simulink model "SquareCartesian_backup"  (R2017b)
settings: Solver=VariableStepAuto  StartTime=0.0  StopTime=50  RelTol=1e-3
PreLoadFcn:
  | config_parameters
model workspace (MAT data in the model file):
  r = 0.11
undefined symbols (not defined in the file): b, sampleTime, X, Y, Z
libraries: sm_lib x127, nesl_utility x20, fl_lib x8, vrlib x4, mobileRoboticsLib x2, simulink x1
(part 1 of 4)
settings Model: Creator=ty  LastModifiedBy=ty
settings DataIOCC: ExternalInput=[r, b]
settings SimMechanicsCC: VisOnUpdateDiagram=on  VisDuringSimulation=on

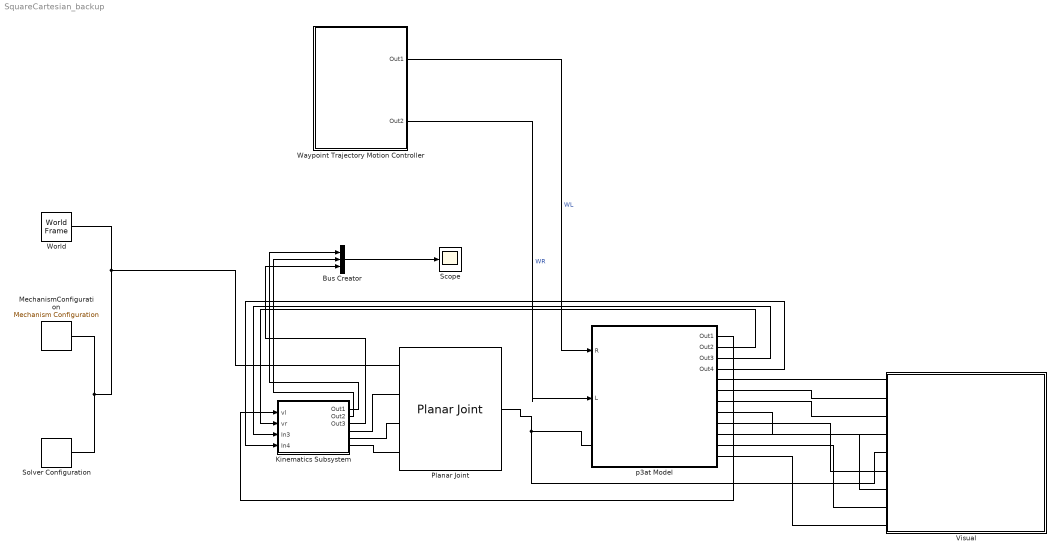
== system SquareCartesian_backup ==
  Bus Creator : BusCreator  Inputs=3
  Kinematics Subsystem : Subsystem
  MechanismConfiguration : sm_lib/Utilities/Mechanism Configuration  UniformGravity=Constant  GravityVector=[0 0 -9.80665]  GravityUnits=m/s^2  LinearizationDelta=0.001
  Planar Joint : sm_lib/Joints/Planar Joint  SenseConstraintForce=off  SenseConstraintForceX=off  SenseConstraintForceY=off  SenseConstraintForceZ=off  SenseConstraintTorque=off  SenseConstraintTorqueX=off  SenseConstraintTorqueY=off  SenseConstraintTorqueZ=off  SenseTotalForce=off  SenseTotalForceX=off  SenseTotalForceY=off  SenseTotalForceZ=off  SenseTotalTorque=off  SenseTotalTorqueX=off  SenseTotalTorqueY=off  SenseTotalTorqueZ=off  CompositeWrenchDir=FollowerOnBase  CompositeWrenchFrame=BaseFrame  PxEquilibriumPosition=0  PxEquilibriumPositionUnits=m  PxSpringStiffness=0  PxSpringStiffnessUnits=N/m  PxDampingCoefficient=0  PxDampingCoefficientUnits=N/(m/s)  PxTorqueActuationMode=ComputedTorque  PxMotionActuationMode=InputMotion  PxSensePosition=off  PxSenseVelocity=off  PxSenseAcceleration=off  PxSenseTorqueForce=off  PxPositionTargetSpecify=on  PxPositionTargetPriority=High  PxPositionTargetValue=0  PxPositionTargetValueUnits=m  PxVelocityTargetSpecify=off  PxVelocityTargetPriority=High  PxVelocityTargetValue=0  PxVelocityTargetValueUnits=m/s  PyEquilibriumPosition=0  PyEquilibriumPositionUnits=m  PySpringStiffness=0  PySpringStiffnessUnits=N/m  PyDampingCoefficient=0  PyDampingCoefficientUnits=N/(m/s)  PyTorqueActuationMode=ComputedTorque  PyMotionActuationMode=InputMotion  PySensePosition=off  PySenseVelocity=off  PySenseAcceleration=off  PySenseTorqueForce=off  PyPositionTargetSpecify=on  PyPositionTargetPriority=High  PyPositionTargetValue=0  PyPositionTargetValueUnits=m  PyVelocityTargetSpecify=off  PyVelocityTargetPriority=High  PyVelocityTargetValue=0  PyVelocityTargetValueUnits=m/s  RzEquilibriumPosition=0  RzEquilibriumPositionUnits=deg  RzSpringStiffness=0  RzSpringStiffnessUnits=N*m/deg  RzDampingCoefficient=0  RzDampingCoefficientUnits=N*m/(deg/s)  RzTorqueActuationMode=ComputedTorque  RzMotionActuationMode=InputMotion  RzSensePosition=off  RzSenseVelocity=off  RzSenseAcceleration=off  RzSenseTorqueForce=off  RzPositionTargetSpecify=on  RzPositionTargetPriority=High  RzPositionTargetValue=0  RzPositionTargetValueUnits=deg  RzVelocityTargetSpecify=off  RzVelocityTargetPriority=High  RzVelocityTargetValue=0  RzVelocityTargetValueUnits=deg/s
  Scope : Scope
  Solver Configuration : nesl_utility/Solver Configuration  PhysicalDomain=network_engine_domain  SubClassName=solver  LeftPortType=input  RightPortType=generic  Accelerate=off  Tones=[]  Harmonics=[]  SimulateNoise=off  Profile=off  UseLocalSampling=off  EnableSwitchedLinearOptims=on  FrequencyDomain=off  UseCCode=off  RelTol=0.001  AbsTol=1e-06  MinStep=1e-09  ToWorkspace=off  RevertToSquareIcSolve=off  NumHomotopyIterations=100  PhasorMode=off  PhasorModeNumHarmonics=1  DoDC=off  ResidualTolerance=1e-09  UseLocalSolver=off  LocalSolverChoice=NE_BACKWARD_EULER_ADVANCER  LocalSolverSampleTime=0.001  DoFixedCost=off  MaxNonlinIter=3  MaxModeIter=2  LinearAlgebra=Sparse  DelaysMemoryBudget=1024  AutomaticFiltering=on  FilteringTimeConstant=0.001
  Visual : Subsystem
  Waypoint Trajectory Motion Controller : Subsystem
  World : sm_lib/Frames and Transforms/World Frame
  p3at Model : Subsystem
  wires:
  p3at Model/1(Out1) -> Kinematics Subsystem/1(vl)
  p3at Model/2(Out2) -> Kinematics Subsystem/2(vr)
  p3at Model/3(Out3) -> Kinematics Subsystem/3(In3)
  p3at Model/4(Out4) -> Kinematics Subsystem/4(In4)
  Kinematics Subsystem/1(Out1) -> Bus Creator/1
  Kinematics Subsystem/2(Out2) -> Bus Creator/2
  Kinematics Subsystem/3(Out3) -> Bus Creator/3
  Bus Creator/1 -> Scope/1
  Waypoint Trajectory Motion Controller/1(Out1) -> p3at Model/1(R)  "WL"
  Waypoint Trajectory Motion Controller/2(Out2) -> p3at Model/2(L)  "WR"
  connections:
  MechanismConfiguration/RConn1 -- Planar Joint/LConn1 -- World/RConn1 -- Solver Configuration/RConn1
  Planar Joint/LConn4 -- Kinematics Subsystem/RConn3
  Kinematics Subsystem/RConn2 -- Planar Joint/LConn3
  Kinematics Subsystem/RConn1 -- Planar Joint/LConn2
  Planar Joint/RConn1 -- Visual/LConn5 -- p3at Model/LConn1
  p3at Model/RConn1 -- Visual/LConn1
  Visual/LConn2 -- p3at Model/RConn2
  Visual/LConn3 -- p3at Model/RConn3
  Visual/LConn4 -- p3at Model/RConn4
  Visual/LConn6 -- p3at Model/RConn5
  Visual/LConn7 -- p3at Model/RConn6
  Visual/LConn8 -- p3at Model/RConn7
  Visual/LConn9 -- p3at Model/RConn8

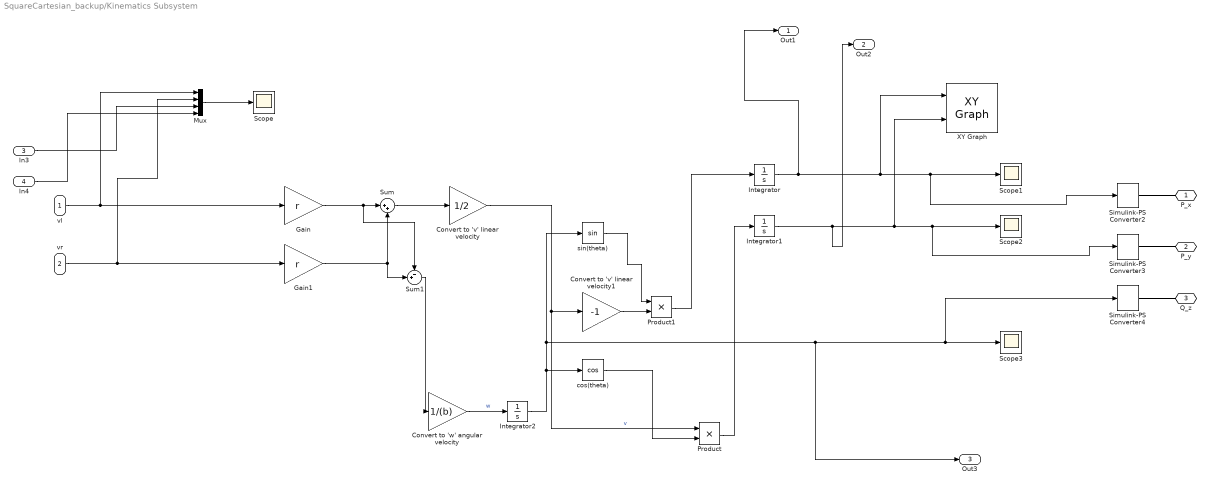
== system SquareCartesian_backup/Kinematics Subsystem ==
  vl : Inport
  vr : Inport  Port=2
  In3 : Inport  Port=3
  In4 : Inport  Port=4
  Convert to 'v' linear velocity : Gain  Gain=1/2
  Convert to 'v' linear velocity1 : Gain  Gain=-1
  Convert to 'w' angular velocity : Gain  Gain=1/(b)
  Gain : Gain  Gain=r
  Gain1 : Gain  Gain=r
  Integrator : Integrator
  Integrator1 : Integrator
  Integrator2 : Integrator
  Mux : Mux
  Product : Product
  Product1 : Product
  Scope{,1..3} (4 alike) : Scope
  Simulink-PS Converter2 : nesl_utility/Simulink-PS Converter  PhysicalDomain=network_engine_domain  SubClassName=ps_input  LeftPortType=input  RightPortType=output  PseudoPeriodic=off  Frequencies=[]  NoiseDistribution=none  NoiseParameters=[]  Unit=1  AffineConversion=off  FilteringAndDerivatives=filter  SimscapeFilterOrder=2  InputFilterTimeConstant=0.01  UdotUserProvided=1
  Simulink-PS Converter3 : nesl_utility/Simulink-PS Converter  PhysicalDomain=network_engine_domain  SubClassName=ps_input  LeftPortType=input  RightPortType=output  PseudoPeriodic=off  Frequencies=[]  NoiseDistribution=none  NoiseParameters=[]  Unit=1  AffineConversion=off  FilteringAndDerivatives=filter  SimscapeFilterOrder=2  InputFilterTimeConstant=0.01  UdotUserProvided=1
  Simulink-PS Converter4 : nesl_utility/Simulink-PS Converter  PhysicalDomain=network_engine_domain  SubClassName=ps_input  LeftPortType=input  RightPortType=output  PseudoPeriodic=off  Frequencies=[]  NoiseDistribution=none  NoiseParameters=[]  Unit=1  AffineConversion=off  FilteringAndDerivatives=filter  SimscapeFilterOrder=2  InputFilterTimeConstant=0.01  UdotUserProvided=1
  Sum : Sum  Inputs=|++
  Sum1 : Sum  Inputs=-+|
  XY Graph : simulink/Sinks/XY Graph  xmin=-10  xmax=10  ymin=-10  ymax=10  st=.05
  cos(theta) : Trigonometry  Operator=cos
  sin(theta) : Trigonometry
  P_x : PMIOPort  Port=1  Side=Right
  P_y : PMIOPort  Port=2  Side=Right
  Q_z : PMIOPort  Port=3  Side=Right
  Out1 : Outport
  Out2 : Outport  Port=2
  Out3 : Outport  Port=3
  wires:
  Convert to 'v' linear velocity1/1 -> Product1/2
  Mux/1 -> Scope/1
  Product/1 -> Integrator1/1
  Product1/1 -> Integrator/1
  vr/1 -> Gain1/1, Mux/2
  vl/1 -> Gain/1, Mux/1
  Convert to 'v' linear velocity/1 -> Product/1, Convert to 'v' linear velocity1/1  "v"
  Sum1/1 -> Convert to 'w' angular velocity/1
  cos(theta)/1 -> Product/2
  sin(theta)/1 -> Product1/1
  Convert to 'w' angular velocity/1 -> Integrator2/1  "w"
  Integrator/1 -> Out1/1, XY Graph/1, Scope1/1, Simulink-PS Converter2/1
  Sum/1 -> Convert to 'v' linear velocity/1
  Gain/1 -> Sum/1, Sum1/1
  Gain1/1 -> Sum1/2, Sum/2
  In3/1 -> Mux/3
  In4/1 -> Mux/4
  Integrator1/1 -> Out2/1, XY Graph/2, Scope2/1, Simulink-PS Converter3/1
  Integrator2/1 -> cos(theta)/1, Scope3/1, Simulink-PS Converter4/1, Out3/1, sin(theta)/1
  connections:
  Simulink-PS Converter3/RConn1 -- P_y/RConn1
  Simulink-PS Converter2/RConn1 -- P_x/RConn1
  Simulink-PS Converter4/RConn1 -- Q_z/RConn1

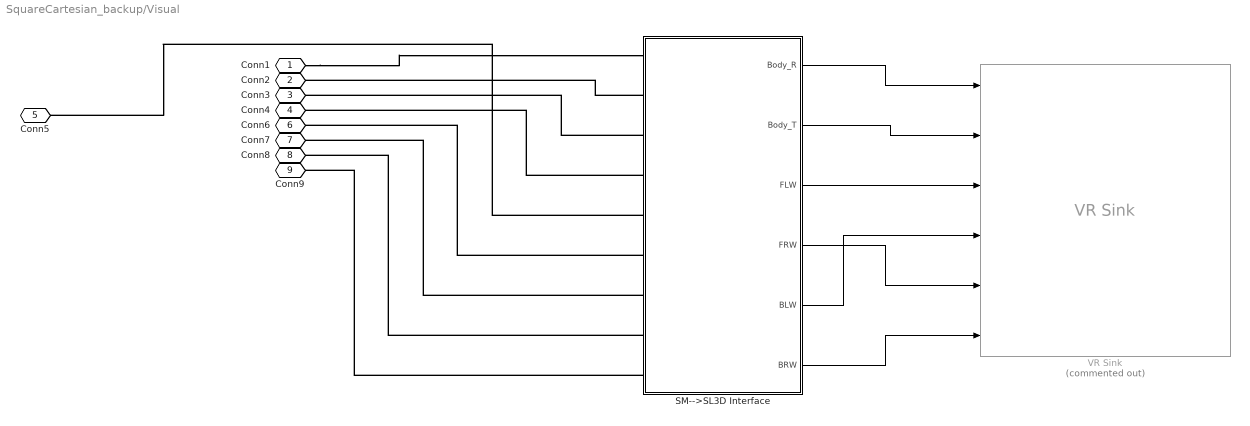
== system SquareCartesian_backup/Visual ==
  SM-->SL3D Interface : Subsystem
  VR Sink : vrlib/VR Sink  Commented=on  InstantiateOnLoad=on  SampleTime=0.1  ViewEnable=on  RemoteChange=off  RemoteView=off  FieldsWritten=URDF_p3original_Transform.rotation.4.1.1.double#URDF_p3original_Transform.translation.3.1.1.double#joint_base_front_left_axle_joint.rotation.4.1.1.double#joint_p3at_back_left_axle_joint.rotation.4.1.1.double#joint_base_front_right_axle_joint.rotation.4.1.1.double#joint_p3at_back_right_axle_joint.rotation.4.1.1.double  WorldFileName=/home/ty/Matlab UGV Simulations/Environments/p3atEnv.wrl  WorldDescription=Pioneer3at Model  AutoView=off  VideoDimensions=[]  AllowVariableSize=off
      settings: SourceProductBaseCode=VR
  Conn1 : PMIOPort  Port=1  Side=Left
  Conn2 : PMIOPort  Port=2  Side=Left
  Conn3 : PMIOPort  Port=3  Side=Left
  Conn4 : PMIOPort  Port=4  Side=Left
  Conn5 : PMIOPort  Port=5  Side=Left
  Conn6 : PMIOPort  Port=6  Side=Left
  Conn7 : PMIOPort  Port=7  Side=Left
  Conn8 : PMIOPort  Port=8  Side=Left
  Conn9 : PMIOPort  Port=9  Side=Left
  wires:
  SM-->SL3D Interface/1(Body_R) -> VR Sink/1
  SM-->SL3D Interface/2(Body_T) -> VR Sink/2
  SM-->SL3D Interface/3(FLW) -> VR Sink/3
  SM-->SL3D Interface/4(FRW) -> VR Sink/5
  SM-->SL3D Interface/5(BLW) -> VR Sink/4
  SM-->SL3D Interface/6(BRW) -> VR Sink/6
  connections:
  SM-->SL3D Interface/LConn5 -- Conn5/RConn1
  SM-->SL3D Interface/LConn3 -- Conn3/RConn1
  Conn1/RConn1 -- SM-->SL3D Interface/LConn1
  SM-->SL3D Interface/LConn7 -- Conn7/RConn1
  SM-->SL3D Interface/LConn2 -- Conn2/RConn1
  SM-->SL3D Interface/LConn6 -- Conn6/RConn1
  SM-->SL3D Interface/LConn8 -- Conn8/RConn1
  SM-->SL3D Interface/LConn4 -- Conn4/RConn1
  SM-->SL3D Interface/LConn9 -- Conn9/RConn1

== system SquareCartesian_backup/Waypoint Trajectory Motion Controller ==
  Differential Drive Inverse Kinematics : Subsystem  AncestorBlock=mobileRoboticsLib/Kinematic Models/Differential Drive/Differential Drive Inverse Kinematics  mask(Differential Drive Inverse Kinematics){wheelRadius=r, wheelBase=b}
      mask prompts: wheelRadius "Wheel Radius [m]"; wheelBase "Wheelbase [m]"
      mask help:
      | Calculates the forward kinematics for a differential drive vehicle.
      |
      | Input: [v; w], the linear (m/s) and angular (rad/s) velocities of the vehicle
      |
      | Output: [wL; wR], the left and right wheel speeds (rad/s)
      mask Help: web('matlab:edit mrsDocDifferentialDrive')
  Differential Drive Simulation : mobileRoboticsLib/Kinematic Models/Differential Drive/Differential Drive Simulation  OverrideUsingVariant=mode==2  wheelRadius=r  wheelBase=b  initX=0  initY=0  initAngle=0  Ts=sampleTime
      settings: SourceProductName=Mobile Robotics Simulation Library
  Mux : Mux  Inputs=2
  Robot Visualizer : mobileRoboticsLib/Environments/Robot Visualizer  Priority=99  robotRadius=.25  showTrajectory=on  hasWaypoints=on  hasLidar=off  sensorOffset=[ 0 0 ]  scanAngles=0  hasObjDetector=off  objDetectorOffset=[ 0, 0 ]  objDetectorAngle=0  objDetectorFOV=0  objDetectorMaxRange=0  objectColors=0  objectMarkers='s'
      settings: SourceProductName=Ground Vehicles Library
  Waypoint Tracking Logic : Stateflow chart  TreatAsAtomicUnit=on
  Waypoints1 : Constant  Value=[0,0; 2,2; -2,2; -2,-2; 2,-2; 2,2; 0,0]
  Out1 : Outport
  Out2 : Outport  Port=2
  wires:
  Differential Drive Inverse Kinematics/3(WR) -> Out1/1
  Differential Drive Inverse Kinematics/2(WL) -> Out2/1
  Differential Drive Simulation/1 -> Waypoint Tracking Logic/1(pose), Robot Visualizer/1  "pose"
  Waypoint Tracking Logic/2(w) -> Mux/2  "w"
  Mux/1 -> Differential Drive Inverse Kinematics/1(vRef)  "vRef"
  Waypoint Tracking Logic/1(v) -> Mux/1  "v"
  Waypoints1/1 -> Robot Visualizer/2, Waypoint Tracking Logic/2(waypoints)
  Differential Drive Inverse Kinematics/1(wheelSpd) -> Differential Drive Simulation/1  "wheelSpeeds"

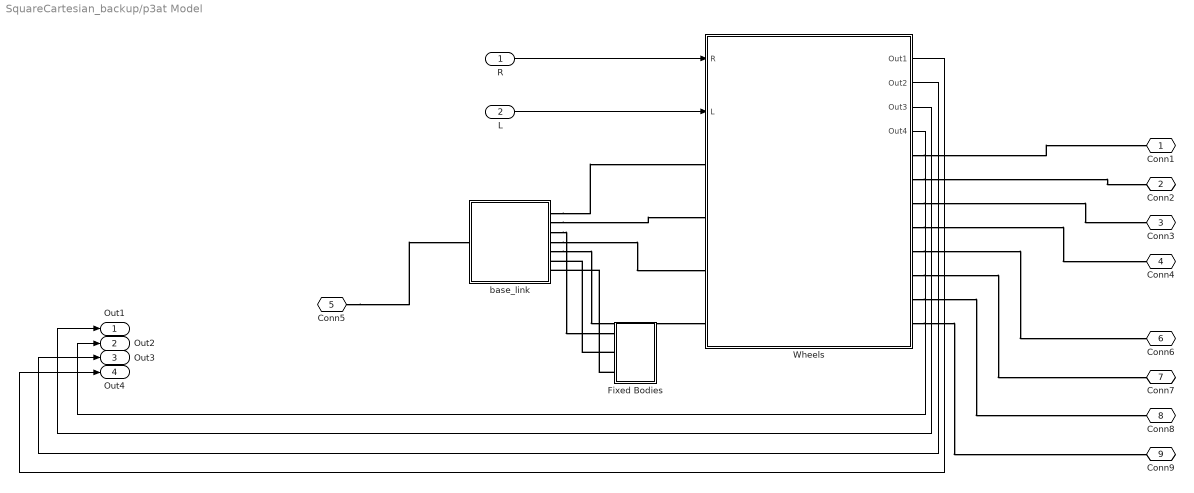
== system SquareCartesian_backup/p3at Model ==
  R : Inport
  L : Inport  Port=2
  Fixed Bodies : Subsystem
  Wheels : Subsystem
  base_link : Subsystem
  Conn1 : PMIOPort  Port=1  Side=Right
  Conn2 : PMIOPort  Port=2  Side=Right
  Conn3 : PMIOPort  Port=3  Side=Right
  Conn4 : PMIOPort  Port=4  Side=Right
  Conn5 : PMIOPort  Port=5  Side=Left
  Conn6 : PMIOPort  Port=6  Side=Right
  Conn7 : PMIOPort  Port=7  Side=Right
  Conn8 : PMIOPort  Port=8  Side=Right
  Conn9 : PMIOPort  Port=9  Side=Right
  Out1 : Outport
  Out2 : Outport  Port=2
  Out3 : Outport  Port=3
  Out4 : Outport  Port=4
  wires:
  Wheels/3(Out3) -> Out1/1
  Wheels/4(Out4) -> Out2/1
  Wheels/2(Out2) -> Out3/1
  Wheels/1(Out1) -> Out4/1
  R/1 -> Wheels/1(R)
  L/1 -> Wheels/2(L)
  connections:
  Conn5/RConn1 -- base_link/LConn1
  base_link/RConn3 -- Fixed Bodies/LConn1
  Fixed Bodies/LConn2 -- base_link/RConn6
  Fixed Bodies/LConn3 -- base_link/RConn7
  Wheels/RConn1 -- Conn1/RConn1
  Wheels/RConn2 -- Conn2/RConn1
  Wheels/RConn3 -- Conn3/RConn1
  Wheels/RConn4 -- Conn4/RConn1
  Wheels/RConn5 -- Conn6/RConn1
  base_link/RConn1 -- Wheels/LConn1
  base_link/RConn2 -- Wheels/LConn2
  Wheels/RConn6 -- Conn7/RConn1
  base_link/RConn4 -- Wheels/LConn3
  base_link/RConn5 -- Wheels/LConn4
  Wheels/RConn7 -- Conn8/RConn1
  Wheels/RConn8 -- Conn9/RConn1

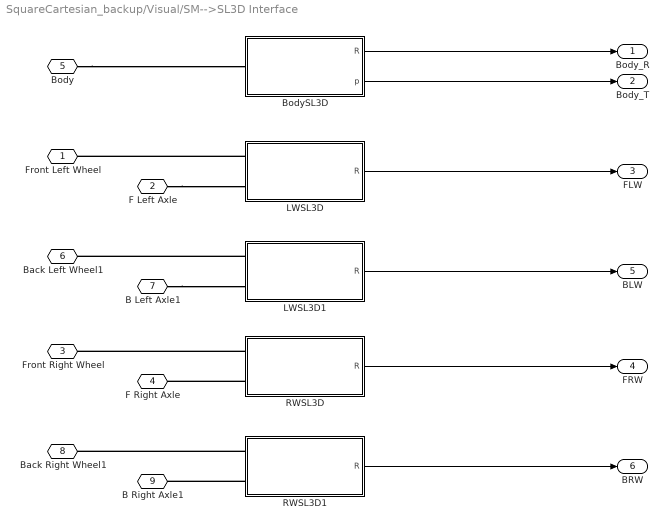
== system SquareCartesian_backup/Visual/SM-->SL3D Interface ==
  "BodySL3D " : Subsystem
  LWSL3D : Subsystem
  LWSL3D1 : Subsystem
  RWSL3D : Subsystem
  RWSL3D1 : Subsystem
  Front Left Wheel : PMIOPort  Port=1  Side=Left
  F Left Axle : PMIOPort  Port=2  Side=Left
  Front Right Wheel : PMIOPort  Port=3  Side=Left
  F Right Axle : PMIOPort  Port=4  Side=Left
  Body : PMIOPort  Port=5  Side=Left
  Back Left Wheel1 : PMIOPort  Port=6  Side=Left
  B Left Axle1 : PMIOPort  Port=7  Side=Left
  Back Right Wheel1 : PMIOPort  Port=8  Side=Left
  B Right Axle1 : PMIOPort  Port=9  Side=Left
  Body_R : Outport
  Body_T : Outport  Port=2
  FLW : Outport  Port=3
  FRW : Outport  Port=4
  BLW : Outport  Port=5
  BRW : Outport  Port=6
  wires:
  "BodySL3D "/1(R) -> Body_R/1
  "BodySL3D "/2(p) -> Body_T/1
  RWSL3D/1(R) -> FRW/1
  LWSL3D/1(R) -> FLW/1
  LWSL3D1/1(R) -> BLW/1
  RWSL3D1/1(R) -> BRW/1
  connections:
  RWSL3D/LConn2 -- F Right Axle/RConn1
  F Left Axle/RConn1 -- LWSL3D/LConn2
  Body/RConn1 -- "BodySL3D "/LConn1
  RWSL3D/LConn1 -- Front Right Wheel/RConn1
  LWSL3D/LConn1 -- Front Left Wheel/RConn1
  B Left Axle1/RConn1 -- LWSL3D1/LConn2
  LWSL3D1/LConn1 -- Back Left Wheel1/RConn1
  RWSL3D1/LConn1 -- Back Right Wheel1/RConn1
  RWSL3D1/LConn2 -- B Right Axle1/RConn1

== system SquareCartesian_backup/Waypoint Trajectory Motion Controller/Differential Drive Inverse Kinematics ==
  vRef : Inport
  Demux : Demux  Outputs=2
  MATLAB Function : MATLAB Function  TreatAsAtomicUnit=on
  Mux : Mux  Inputs=2
  wheelSpd : Outport
  WL : Outport  Port=2
  WR : Outport  Port=3
  wires:
  MATLAB Function/1(wL) -> WL/1, Mux/1  "wL"
  MATLAB Function/2(wR) -> WR/1, Mux/2  "wR"
  Mux/1 -> wheelSpd/1
  vRef/1 -> Demux/1
  Demux/1 -> MATLAB Function/1(v)  "v"
  Demux/2 -> MATLAB Function/2(w)  "w"

== system SquareCartesian_backup/p3at Model/Fixed Bodies ==
  Sonar Arrays : Subsystem
  Top Plate : Subsystem
  Conn1 : PMIOPort  Port=1  Side=Left
  Conn2 : PMIOPort  Port=2  Side=Left
  Conn3 : PMIOPort  Port=3  Side=Left
  connections:
  Conn1/RConn1 -- Top Plate/LConn1
  Sonar Arrays/LConn1 -- Conn2/RConn1
  Sonar Arrays/LConn2 -- Conn3/RConn1

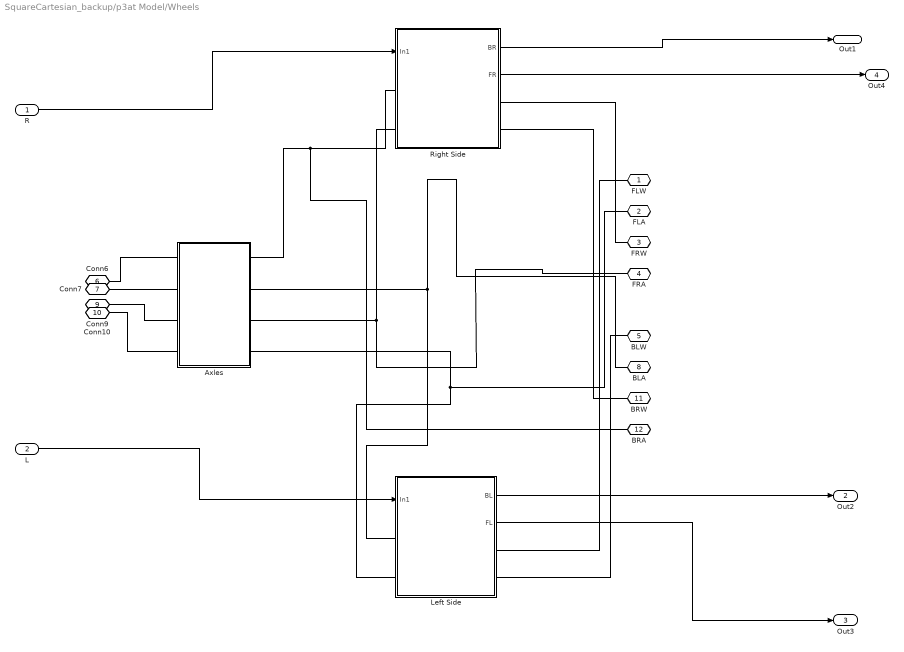
== system SquareCartesian_backup/p3at Model/Wheels ==
  R : Inport
  L : Inport  Port=2
  Axles : Subsystem
  Left Side : Subsystem
  Right Side : Subsystem
  FLW : PMIOPort  Port=1  Side=Right
  FLA : PMIOPort  Port=2  Side=Right
  FRW : PMIOPort  Port=3  Side=Right
  FRA : PMIOPort  Port=4  Side=Right
  BLW : PMIOPort  Port=5  Side=Right
  Conn6 : PMIOPort  Port=6  Side=Left
  Conn7 : PMIOPort  Port=7  Side=Left
  BLA : PMIOPort  Port=8  Side=Right
  Conn9 : PMIOPort  Port=9  Side=Left
  Conn10 : PMIOPort  Port=10  Side=Left
  BRW : PMIOPort  Port=11  Side=Right
  BRA : PMIOPort  Port=12  Side=Right
  Out1 : Outport
  Out2 : Outport  Port=2
  Out3 : Outport  Port=3
  Out4 : Outport  Port=4
  wires:
  R/1 -> Right Side/1(In1)
  Right Side/1(BR) -> Out1/1
  Right Side/2(FR) -> Out4/1
  L/1 -> Left Side/1(In1)
  Left Side/1(BL) -> Out2/1
  Left Side/2(FL) -> Out3/1
  connections:
  FLA/RConn1 -- Left Side/LConn2 -- Axles/RConn4
  FRA/RConn1 -- Axles/RConn3 -- Right Side/LConn2
  BLA/RConn1 -- Left Side/LConn1 -- Axles/RConn2
  Conn6/RConn1 -- Axles/LConn1
  Conn7/RConn1 -- Axles/LConn2
  Axles/LConn3 -- Conn9/RConn1
  Axles/LConn4 -- Conn10/RConn1
  Axles/RConn1 -- Right Side/LConn1 -- BRA/RConn1
  FRW/RConn1 -- Right Side/RConn1
  BRW/RConn1 -- Right Side/RConn2
  Left Side/RConn1 -- FLW/RConn1
  BLW/RConn1 -- Left Side/RConn2

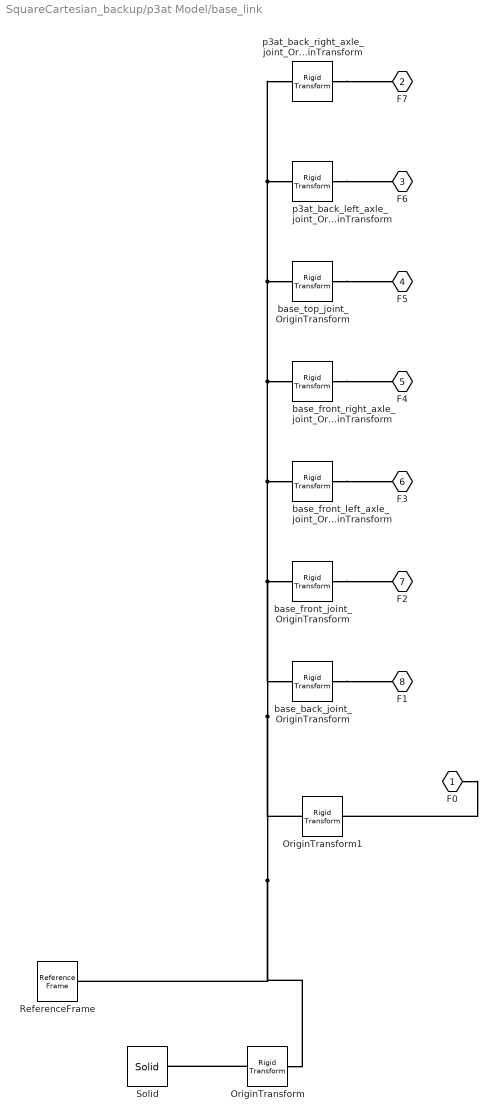
== system SquareCartesian_backup/p3at Model/base_link ==
  OriginTransform : sm_lib/Frames and Transforms/Rigid Transform  TranslationMethod=Cartesian  TranslationStandardOffset=0  TranslationLengthUnit=m  TranslationStandardAxis=+Z  TranslationCartesianOffset=[0, 0, -0.177]  TranslationROffset=0  TranslationROffsetUnits=m  TranslationZOffset=0  TranslationZOffsetUnits=m  TranslationThetaOffset=0  TranslationThetaOffsetUnits=deg  RotationMethod=RotationSequence  RotationAngleUnits=deg  RotationStandardAxis=+Z  RotationAngle=0.0  RotationArbitraryAxis=[0 0 1]  FollAlignAxisA=+X  BaseAlignAxisA=+Y  FollAlignAxisB=+Y  BaseAlignAxisB=+Z  RotationSequenceAxes=BaseAxes  RotationSequence=XYZ  RotationSequenceAngles=[0, 0, 0]  RotationSequenceAnglesUnits=rad  RotationMatrix=[1 0 0; 0 1 0; 0 0 1]
  OriginTransform1 : sm_lib/Frames and Transforms/Rigid Transform  TranslationMethod=Cartesian  TranslationStandardOffset=0  TranslationLengthUnit=m  TranslationStandardAxis=+Z  TranslationCartesianOffset=[0, 0, -0.177]  TranslationROffset=0  TranslationROffsetUnits=m  TranslationZOffset=0  TranslationZOffsetUnits=m  TranslationThetaOffset=0  TranslationThetaOffsetUnits=deg  RotationMethod=StandardAxis  RotationAngleUnits=deg  RotationStandardAxis=+Z  RotationAngle=90.0  RotationArbitraryAxis=[0 0 1]  FollAlignAxisA=+X  BaseAlignAxisA=+Y  FollAlignAxisB=+Y  BaseAlignAxisB=+Z  RotationSequenceAxes=BaseAxes  RotationSequence=XYZ  RotationSequenceAngles=[0, 0, 0]  RotationSequenceAnglesUnits=rad  RotationMatrix=[1 0 0; 0 1 0; 0 0 1]
  ReferenceFrame : sm_lib/Frames and Transforms/Reference Frame
  Solid : sm_lib/Body Elements/Solid  InertiaType=Custom  Mass=21.5  MassUnits=kg  CenterOfMass=[0, 0, 0]  CenterOfMassUnits=m  MomentsOfInertia=[0.3338, 0.4783, 0.3338]  MomentsOfInertiaUnits=kg*m^2  ProductsOfInertia=[0, 0, 0]  ProductsOfInertiaUnits=kg*m^2  DensityBased=on  Density=1000  DensityUnits=kg/(m^3)  DoExposeReferenceFrame=on  SerializedFrames=<Frames/>  GraphicType=FromGeometry  MarkerShape=Sphere  MarkerSize=10  MarkerSizeUnits=m  GraphicVisPropType=SimpleVisualProperties  GraphicDiffuseColor=[0.851, 0, 0]  GraphicSpecularColor=[0.5 0.5 0.5 1.0]  GraphicAmbientColor=[0.15 0.15 0.15 1.0]  GraphicEmissiveColor=[0.0 0.0 0.0 1.0]  GraphicShininess=75  GraphicOpacity=1  GeometryShape=FromFile  RectangleSize=[1 1]  RectangleSizeUnits=m  BrickDimensions=[1 1 1]  BrickDimensionUnits=m  CylinderRadius=1  CylinderRadiusUnits=m  CylinderLength=1  CylinderLengthUnits=m  SphereRadius=1  SphereRadiusUnits=m  EllipsoidRadii=[1 1 1]  EllipsoidRadiiUnits=m  ExtrusionCrossSection=[1 1; -1 1; -1 -1; 1 -1]  ExtrusionCrossSectionUnits=m  ExtrusionLength=1  ExtrusionLengthUnits=m  PolygonNumSides=3  PolygonOuterRadius=1  PolygonOuterRadiusUnits=m  ExtGeomFileType=STL  ExtGeomFileName=/home/ty/Matlab UGV Simulations/Models/p3at_meshes/chassis.stl  ExtGeomFileUnits=m  RevolutionCrossSection=[1 1; 1 -1; 2 -1; 2 1]  RevolutionCrossSectionUnits=m  RevolutionExtent=Full  RevolutionAngle=180  RevolutionAngleUnits=deg
  base_back_joint_OriginTransform : sm_lib/Frames and Transforms/Rigid Transform  TranslationMethod=Cartesian  TranslationStandardOffset=0  TranslationLengthUnit=m  TranslationStandardAxis=+Z  TranslationCartesianOffset=[-0.187, 0, 0.247]  TranslationROffset=0  TranslationROffsetUnits=m  TranslationZOffset=0  TranslationZOffsetUnits=m  TranslationThetaOffset=0  TranslationThetaOffsetUnits=deg  RotationMethod=RotationSequence  RotationAngleUnits=deg  RotationStandardAxis=+Z  RotationAngle=0.0  RotationArbitraryAxis=[0 0 1]  FollAlignAxisA=+X  BaseAlignAxisA=+Y  FollAlignAxisB=+Y  BaseAlignAxisB=+Z  RotationSequenceAxes=BaseAxes  RotationSequence=XYZ  RotationSequenceAngles=[0, 0, 0]  RotationSequenceAnglesUnits=rad  RotationMatrix=[1 0 0; 0 1 0; 0 0 1]
  base_front_joint_OriginTransform : sm_lib/Frames and Transforms/Rigid Transform  TranslationMethod=Cartesian  TranslationStandardOffset=0  TranslationLengthUnit=m  TranslationStandardAxis=+Z  TranslationCartesianOffset=[0.193, 0, 0.25]  TranslationROffset=0  TranslationROffsetUnits=m  TranslationZOffset=0  TranslationZOffsetUnits=m  TranslationThetaOffset=0  TranslationThetaOffsetUnits=deg  RotationMethod=RotationSequence  RotationAngleUnits=deg  RotationStandardAxis=+Z  RotationAngle=0.0  RotationArbitraryAxis=[0 0 1]  FollAlignAxisA=+X  BaseAlignAxisA=+Y  FollAlignAxisB=+Y  BaseAlignAxisB=+Z  RotationSequenceAxes=BaseAxes  RotationSequence=XYZ  RotationSequenceAngles=[0, 0, 0]  RotationSequenceAnglesUnits=rad  RotationMatrix=[1 0 0; 0 1 0; 0 0 1]
  base_front_left_axle_joint_OriginTransform : sm_lib/Frames and Transforms/Rigid Transform  TranslationMethod=Cartesian  TranslationStandardOffset=0  TranslationLengthUnit=m  TranslationStandardAxis=+Z  TranslationCartesianOffset=[0.135, 0.156, 0.111]  TranslationROffset=0  TranslationROffsetUnits=m  TranslationZOffset=0  TranslationZOffsetUnits=m  TranslationThetaOffset=0  TranslationThetaOffsetUnits=deg  RotationMethod=RotationSequence  RotationAngleUnits=deg  RotationStandardAxis=+Z  RotationAngle=0.0  RotationArbitraryAxis=[0 0 1]  FollAlignAxisA=+X  BaseAlignAxisA=+Y  FollAlignAxisB=+Y  BaseAlignAxisB=+Z  RotationSequenceAxes=BaseAxes  RotationSequence=XYZ  RotationSequenceAngles=[0, 0, 0]  RotationSequenceAnglesUnits=rad  RotationMatrix=[1 0 0; 0 1 0; 0 0 1]
  base_front_right_axle_joint_OriginTransform : sm_lib/Frames and Transforms/Rigid Transform  TranslationMethod=Cartesian  TranslationStandardOffset=0  TranslationLengthUnit=m  TranslationStandardAxis=+Z  TranslationCartesianOffset=[0.135, -0.156, 0.111]  TranslationROffset=0  TranslationROffsetUnits=m  TranslationZOffset=0  TranslationZOffsetUnits=m  TranslationThetaOffset=0  TranslationThetaOffsetUnits=deg  RotationMethod=RotationSequence  RotationAngleUnits=deg  RotationStandardAxis=+Z  RotationAngle=0.0  RotationArbitraryAxis=[0 0 1]  FollAlignAxisA=+X  BaseAlignAxisA=+Y  FollAlignAxisB=+Y  BaseAlignAxisB=+Z  RotationSequenceAxes=BaseAxes  RotationSequence=XYZ  RotationSequenceAngles=[0, 0, 0]  RotationSequenceAnglesUnits=rad  RotationMatrix=[1 0 0; 0 1 0; 0 0 1]
  base_top_joint_OriginTransform : sm_lib/Frames and Transforms/Rigid Transform  TranslationMethod=Cartesian  TranslationStandardOffset=0  TranslationLengthUnit=m  TranslationStandardAxis=+Z  TranslationCartesianOffset=[0.003, 0, 0.274]  TranslationROffset=0  TranslationROffsetUnits=m  TranslationZOffset=0  TranslationZOffsetUnits=m  TranslationThetaOffset=0  TranslationThetaOffsetUnits=deg  RotationMethod=RotationSequence  RotationAngleUnits=deg  RotationStandardAxis=+Z  RotationAngle=0.0  RotationArbitraryAxis=[0 0 1]  FollAlignAxisA=+X  BaseAlignAxisA=+Y  FollAlignAxisB=+Y  BaseAlignAxisB=+Z  RotationSequenceAxes=BaseAxes  RotationSequence=XYZ  RotationSequenceAngles=[0, 0, 0]  RotationSequenceAnglesUnits=rad  RotationMatrix=[1 0 0; 0 1 0; 0 0 1]
  p3at_back_left_axle_joint_OriginTransform : sm_lib/Frames and Transforms/Rigid Transform  TranslationMethod=Cartesian  TranslationStandardOffset=0  TranslationLengthUnit=m  TranslationStandardAxis=+Z  TranslationCartesianOffset=[-0.134, 0.156, 0.111]  TranslationROffset=0  TranslationROffsetUnits=m  TranslationZOffset=0  TranslationZOffsetUnits=m  TranslationThetaOffset=0  TranslationThetaOffsetUnits=deg  RotationMethod=RotationSequence  RotationAngleUnits=deg  RotationStandardAxis=+Z  RotationAngle=0.0  RotationArbitraryAxis=[0 0 1]  FollAlignAxisA=+X  BaseAlignAxisA=+Y  FollAlignAxisB=+Y  BaseAlignAxisB=+Z  RotationSequenceAxes=BaseAxes  RotationSequence=XYZ  RotationSequenceAngles=[0, 0, 0]  RotationSequenceAnglesUnits=rad  RotationMatrix=[1 0 0; 0 1 0; 0 0 1]
  p3at_back_right_axle_joint_OriginTransform : sm_lib/Frames and Transforms/Rigid Transform  TranslationMethod=Cartesian  TranslationStandardOffset=0  TranslationLengthUnit=m  TranslationStandardAxis=+Z  TranslationCartesianOffset=[-0.134, -0.156, 0.111]  TranslationROffset=0  TranslationROffsetUnits=m  TranslationZOffset=0  TranslationZOffsetUnits=m  TranslationThetaOffset=0  TranslationThetaOffsetUnits=deg  RotationMethod=ArbitraryAxis  RotationAngleUnits=rad  RotationStandardAxis=+Z  RotationAngle=0  RotationArbitraryAxis=[-0.57735026918962573 -0.57735026918962584 0.57735026918962573]  FollAlignAxisA=+X  BaseAlignAxisA=+Y  FollAlignAxisB=+Y  BaseAlignAxisB=+Z  RotationSequenceAxes=BaseAxes  RotationSequence=XYZ  RotationSequenceAngles=[0, 0, 0]  RotationSequenceAnglesUnits=rad  RotationMatrix=[1 0 0; 0 1 0; 0 0 1]
  F0 : PMIOPort  Port=1  Side=Left
  F7 : PMIOPort  Port=2  Side=Right
  F6 : PMIOPort  Port=3  Side=Right
  F5 : PMIOPort  Port=4  Side=Right
  F4 : PMIOPort  Port=5  Side=Right
  F3 : PMIOPort  Port=6  Side=Right
  F2 : PMIOPort  Port=7  Side=Right
  F1 : PMIOPort  Port=8  Side=Right
  connections:
  OriginTransform1/LConn1 -- OriginTransform/RConn1 -- ReferenceFrame/RConn1 -- base_back_joint_OriginTransform/LConn1 -- p3at_back_left_axle_joint_OriginTransform/LConn1 -- p3at_back_right_axle_joint_OriginTransform/LConn1 -- base_top_joint_OriginTransform/LConn1 -- base_front_right_axle_joint_OriginTransform/LConn1 -- base_front_left_axle_joint_OriginTransform/LConn1 -- base_front_joint_OriginTransform/LConn1
  base_back_joint_OriginTransform/RConn1 -- F1/RConn1
  base_front_joint_OriginTransform/RConn1 -- F2/RConn1
  base_front_left_axle_joint_OriginTransform/RConn1 -- F3/RConn1
  base_front_right_axle_joint_OriginTransform/RConn1 -- F4/RConn1
  base_top_joint_OriginTransform/RConn1 -- F5/RConn1
  p3at_back_left_axle_joint_OriginTransform/RConn1 -- F6/RConn1
  p3at_back_right_axle_joint_OriginTransform/RConn1 -- F7/RConn1
  OriginTransform/LConn1 -- Solid/RConn1
  F0/RConn1 -- OriginTransform1/RConn1

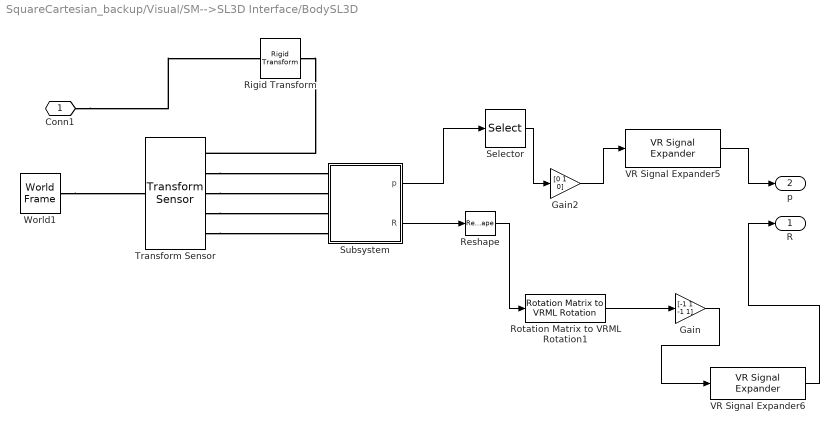
== system SquareCartesian_backup/Visual/SM-->SL3D Interface/BodySL3D  ==
  Gain : Gain  Gain=[-1 1 -1 1]  SaturateOnIntegerOverflow=on  OutDataTypeStr=Inherit: Same as input  ParamDataTypeStr=Inherit: Same as input
  Gain2 : Gain  Gain=[0 1 0]  SaturateOnIntegerOverflow=on  OutDataTypeStr=Inherit: Same as input  ParamDataTypeStr=Inherit: Same as input
  Reshape : Reshape  OutputDimensionality=Customize  OutputDimensions=[3 3]
  Rigid Transform : sm_lib/Frames and Transforms/Rigid Transform  TranslationMethod=StandardAxis  TranslationStandardOffset=0  TranslationLengthUnit=m  TranslationStandardAxis=+Z  TranslationCartesianOffset=[0 0 0]  TranslationROffset=0  TranslationROffsetUnits=m  TranslationZOffset=0  TranslationZOffsetUnits=m  TranslationThetaOffset=0  TranslationThetaOffsetUnits=deg  RotationMethod=StandardAxis  RotationAngleUnits=deg  RotationStandardAxis=-X  RotationAngle=90  RotationArbitraryAxis=[1 0 0]  FollAlignAxisA=+X  BaseAlignAxisA=+Y  FollAlignAxisB=+Y  BaseAlignAxisB=+Z  RotationSequenceAxes=FollowerAxes  RotationSequence=XYX  RotationSequenceAngles=[0 0 0]  RotationSequenceAnglesUnits=deg  RotationMatrix=[1 0 0; 0 1 0; 0 0 1]
  Rotation Matrix to VRML Rotation1 : vrlib/Utilities/Rotation Matrix to VRML Rotation  maxzero=1e-12
      settings: SourceProductName=Simulink 3D Animation  SourceProductBaseCode=VR
  Selector : Selector  InputPortWidth=3  IndexOptions=Index vector (dialog)  Indices=[2 1 3]  OutputSizes=1
  Subsystem : Subsystem
  Transform Sensor : sm_lib/Frames and Transforms/Transform Sensor  MeasurementFrame=World  SenseAngle=off  SenseAxis=off  SenseAngle1=off  SenseAngle2=off  SenseAngle3=off  SenseQ=off  SenseR=on  SenseOmegaX=off  SenseOmegaY=off  SenseOmegaZ=off  SenseOmega1=off  SenseOmega2=off  SenseOmega3=off  SenseQDot=off  SenseRDot=off  SenseAlphaX=off  SenseAlphaY=off  SenseAlphaZ=off  SenseAlpha1=off  SenseAlpha2=off  SenseAlpha3=off  SenseQDDot=off  SenseRDDot=off  SenseX=on  SenseY=on  SenseZ=on  SenseRad=off  SenseAzim=off  SenseDist=off  SenseInc=off  SenseXDot=off  SenseYDot=off  SenseZDot=off  SenseRadDot=off  SenseAzimDot=off  SenseDistDot=off  SenseIncDot=off  SenseXDDot=off  SenseYDDot=off  SenseZDDot=off  SenseRadDDot=off  SenseAzimDDot=off  SenseDistDDot=off  SenseIncDDot=off
  VR Signal Expander5 : vrlib/VR Signal Expander  outwidth=3  outidx=[3 1 2]
      settings: SourceProductName=Simulink 3D Animation  SourceProductBaseCode=VR
  VR Signal Expander6 : vrlib/VR Signal Expander  outwidth=4  outidx=[1 3 2 4]
      settings: SourceProductName=Simulink 3D Animation  SourceProductBaseCode=VR
  World1 : sm_lib/Frames and Transforms/World Frame
  Conn1 : PMIOPort  Port=1  Side=Left
  R : Outport
  p : Outport  Port=2
  wires:
  Subsystem/2(R) -> Reshape/1
  Reshape/1 -> Rotation Matrix to VRML Rotation1/1
  Gain2/1 -> VR Signal Expander5/1
  VR Signal Expander5/1 -> p/1
  Rotation Matrix to VRML Rotation1/1 -> Gain/1
  Gain/1 -> VR Signal Expander6/1
  VR Signal Expander6/1 -> R/1
  Subsystem/1(p) -> Selector/1
  Selector/1 -> Gain2/1
  connections:
  Transform Sensor/RConn4 -- Subsystem/LConn3
  Transform Sensor/RConn5 -- Subsystem/LConn4
  Transform Sensor/RConn2 -- Subsystem/LConn1
  Transform Sensor/RConn3 -- Subsystem/LConn2
  World1/RConn1 -- Transform Sensor/LConn1
  Conn1/RConn1 -- Rigid Transform/LConn1
  Rigid Transform/RConn1 -- Transform Sensor/RConn1

== system SquareCartesian_backup/Visual/SM-->SL3D Interface/LWSL3D ==
  Integrator : Integrator
  Subsystem : Subsystem
  Transform Sensor1 : sm_lib/Frames and Transforms/Transform Sensor  MeasurementFrame=Base  SenseAngle=off  SenseAxis=off  SenseAngle1=off  SenseAngle2=off  SenseAngle3=off  SenseQ=off  SenseR=off  SenseOmegaX=off  SenseOmegaY=off  SenseOmegaZ=on  SenseOmega1=off  SenseOmega2=off  SenseOmega3=off  SenseQDot=off  SenseRDot=off  SenseAlphaX=off  SenseAlphaY=off  SenseAlphaZ=off  SenseAlpha1=off  SenseAlpha2=off  SenseAlpha3=off  SenseQDDot=off  SenseRDDot=off  SenseX=off  SenseY=off  SenseZ=off  SenseRad=off  SenseAzim=off  SenseDist=off  SenseInc=off  SenseXDot=off  SenseYDot=off  SenseZDot=off  SenseRadDot=off  SenseAzimDot=off  SenseDistDot=off  SenseIncDot=off  SenseXDDot=off  SenseYDDot=off  SenseZDDot=off  SenseRadDDot=off  SenseAzimDDot=off  SenseDistDDot=off  SenseIncDDot=off
  Vector Concatenate : Concatenate
  Y Rotation in VRML : Constant  Value=[0 1 0]
  Conn1 : PMIOPort  Port=1  Side=Left
  Conn2 : PMIOPort  Port=2  Side=Left
  R : Outport
  wires:
  Vector Concatenate/1 -> R/1
  Y Rotation in VRML/1 -> Vector Concatenate/1
  Subsystem/1(Omega_z) -> Integrator/1
  Integrator/1 -> Vector Concatenate/2
  connections:
  Subsystem/LConn1 -- Transform Sensor1/RConn2
  Conn2/RConn1 -- Transform Sensor1/LConn1
  Conn1/RConn1 -- Transform Sensor1/RConn1

== system SquareCartesian_backup/Visual/SM-->SL3D Interface/LWSL3D1 ==
  Integrator : Integrator
  Subsystem : Subsystem
  Transform Sensor1 : sm_lib/Frames and Transforms/Transform Sensor  MeasurementFrame=Base  SenseAngle=off  SenseAxis=off  SenseAngle1=off  SenseAngle2=off  SenseAngle3=off  SenseQ=off  SenseR=off  SenseOmegaX=off  SenseOmegaY=off  SenseOmegaZ=on  SenseOmega1=off  SenseOmega2=off  SenseOmega3=off  SenseQDot=off  SenseRDot=off  SenseAlphaX=off  SenseAlphaY=off  SenseAlphaZ=off  SenseAlpha1=off  SenseAlpha2=off  SenseAlpha3=off  SenseQDDot=off  SenseRDDot=off  SenseX=off  SenseY=off  SenseZ=off  SenseRad=off  SenseAzim=off  SenseDist=off  SenseInc=off  SenseXDot=off  SenseYDot=off  SenseZDot=off  SenseRadDot=off  SenseAzimDot=off  SenseDistDot=off  SenseIncDot=off  SenseXDDot=off  SenseYDDot=off  SenseZDDot=off  SenseRadDDot=off  SenseAzimDDot=off  SenseDistDDot=off  SenseIncDDot=off
  Vector Concatenate : Concatenate
  Y Rotation in VRML : Constant  Value=[0 1 0]
  Conn1 : PMIOPort  Port=1  Side=Left
  Conn2 : PMIOPort  Port=2  Side=Left
  R : Outport
  wires:
  Vector Concatenate/1 -> R/1
  Y Rotation in VRML/1 -> Vector Concatenate/1
  Subsystem/1(Omega_z) -> Integrator/1
  Integrator/1 -> Vector Concatenate/2
  connections:
  Subsystem/LConn1 -- Transform Sensor1/RConn2
  Conn2/RConn1 -- Transform Sensor1/LConn1
  Conn1/RConn1 -- Transform Sensor1/RConn1

== system SquareCartesian_backup/Visual/SM-->SL3D Interface/RWSL3D ==
  Gain : Gain  Gain=-1
  Integrator : Integrator
  Subsystem : Subsystem
  Transform Sensor1 : sm_lib/Frames and Transforms/Transform Sensor  MeasurementFrame=Base  SenseAngle=off  SenseAxis=off  SenseAngle1=off  SenseAngle2=off  SenseAngle3=off  SenseQ=off  SenseR=off  SenseOmegaX=off  SenseOmegaY=off  SenseOmegaZ=on  SenseOmega1=off  SenseOmega2=off  SenseOmega3=off  SenseQDot=off  SenseRDot=off  SenseAlphaX=off  SenseAlphaY=off  SenseAlphaZ=off  SenseAlpha1=off  SenseAlpha2=off  SenseAlpha3=off  SenseQDDot=off  SenseRDDot=off  SenseX=off  SenseY=off  SenseZ=off  SenseRad=off  SenseAzim=off  SenseDist=off  SenseInc=off  SenseXDot=off  SenseYDot=off  SenseZDot=off  SenseRadDot=off  SenseAzimDot=off  SenseDistDot=off  SenseIncDot=off  SenseXDDot=off  SenseYDDot=off  SenseZDDot=off  SenseRadDDot=off  SenseAzimDDot=off  SenseDistDDot=off  SenseIncDDot=off
  Vector Concatenate : Concatenate
  Y Rotation in VRML : Constant  Value=[0 1 0]
  Conn1 : PMIOPort  Port=1  Side=Left
  Conn2 : PMIOPort  Port=2  Side=Left
  R : Outport
  wires:
  Gain/1 -> Integrator/1
  Integrator/1 -> Vector Concatenate/2
  Subsystem/1(Omega_z) -> Gain/1
  Y Rotation in VRML/1 -> Vector Concatenate/1
  Vector Concatenate/1 -> R/1
  connections:
  Conn1/RConn1 -- Transform Sensor1/RConn1
  Conn2/RConn1 -- Transform Sensor1/LConn1
  Subsystem/LConn1 -- Transform Sensor1/RConn2

== system SquareCartesian_backup/Visual/SM-->SL3D Interface/RWSL3D1 ==
  Gain : Gain  Gain=-1
  Integrator : Integrator
  Subsystem : Subsystem
  Transform Sensor1 : sm_lib/Frames and Transforms/Transform Sensor  MeasurementFrame=Base  SenseAngle=off  SenseAxis=off  SenseAngle1=off  SenseAngle2=off  SenseAngle3=off  SenseQ=off  SenseR=off  SenseOmegaX=off  SenseOmegaY=off  SenseOmegaZ=on  SenseOmega1=off  SenseOmega2=off  SenseOmega3=off  SenseQDot=off  SenseRDot=off  SenseAlphaX=off  SenseAlphaY=off  SenseAlphaZ=off  SenseAlpha1=off  SenseAlpha2=off  SenseAlpha3=off  SenseQDDot=off  SenseRDDot=off  SenseX=off  SenseY=off  SenseZ=off  SenseRad=off  SenseAzim=off  SenseDist=off  SenseInc=off  SenseXDot=off  SenseYDot=off  SenseZDot=off  SenseRadDot=off  SenseAzimDot=off  SenseDistDot=off  SenseIncDot=off  SenseXDDot=off  SenseYDDot=off  SenseZDDot=off  SenseRadDDot=off  SenseAzimDDot=off  SenseDistDDot=off  SenseIncDDot=off
  Vector Concatenate : Concatenate
  Y Rotation in VRML : Constant  Value=[0 1 0]
  Conn1 : PMIOPort  Port=1  Side=Left
  Conn2 : PMIOPort  Port=2  Side=Left
  R : Outport
  wires:
  Gain/1 -> Integrator/1
  Integrator/1 -> Vector Concatenate/2
  Subsystem/1(Omega_z) -> Gain/1
  Y Rotation in VRML/1 -> Vector Concatenate/1
  Vector Concatenate/1 -> R/1
  connections:
  Conn1/RConn1 -- Transform Sensor1/RConn1
  Conn2/RConn1 -- Transform Sensor1/LConn1
  Subsystem/LConn1 -- Transform Sensor1/RConn2

== system SquareCartesian_backup/p3at Model/Fixed Bodies/Sonar Arrays ==
  back_sonar : Subsystem
  base_back_joint : sm_lib/Joints/Weld Joint  SenseConstraintForce=off  SenseConstraintForceX=off  SenseConstraintForceY=off  SenseConstraintForceZ=off  SenseConstraintTorque=off  SenseConstraintTorqueX=off  SenseConstraintTorqueY=off  SenseConstraintTorqueZ=off  SenseTotalForce=off  SenseTotalForceX=off  SenseTotalForceY=off  SenseTotalForceZ=off  SenseTotalTorque=off  SenseTotalTorqueX=off  SenseTotalTorqueY=off  SenseTotalTorqueZ=off  CompositeWrenchDir=FollowerOnBase  CompositeWrenchFrame=BaseFrame
  base_front_joint : sm_lib/Joints/Weld Joint  SenseConstraintForce=off  SenseConstraintForceX=off  SenseConstraintForceY=off  SenseConstraintForceZ=off  SenseConstraintTorque=off  SenseConstraintTorqueX=off  SenseConstraintTorqueY=off  SenseConstraintTorqueZ=off  SenseTotalForce=off  SenseTotalForceX=off  SenseTotalForceY=off  SenseTotalForceZ=off  SenseTotalTorque=off  SenseTotalTorqueX=off  SenseTotalTorqueY=off  SenseTotalTorqueZ=off  CompositeWrenchDir=FollowerOnBase  CompositeWrenchFrame=BaseFrame
  front_sonar : Subsystem
  Conn1 : PMIOPort  Port=1  Side=Left
  Conn2 : PMIOPort  Port=2  Side=Left
  connections:
  back_sonar/LConn1 -- base_back_joint/RConn1
  base_front_joint/RConn1 -- front_sonar/LConn1
  base_front_joint/LConn1 -- Conn1/RConn1
  base_back_joint/LConn1 -- Conn2/RConn1

== system SquareCartesian_backup/p3at Model/Fixed Bodies/Top Plate ==
  base_top_joint : sm_lib/Joints/Weld Joint  SenseConstraintForce=off  SenseConstraintForceX=off  SenseConstraintForceY=off  SenseConstraintForceZ=off  SenseConstraintTorque=off  SenseConstraintTorqueX=off  SenseConstraintTorqueY=off  SenseConstraintTorqueZ=off  SenseTotalForce=off  SenseTotalForceX=off  SenseTotalForceY=off  SenseTotalForceZ=off  SenseTotalTorque=off  SenseTotalTorqueX=off  SenseTotalTorqueY=off  SenseTotalTorqueZ=off  CompositeWrenchDir=FollowerOnBase  CompositeWrenchFrame=BaseFrame
  top_plate : Subsystem
  Conn1 : PMIOPort  Port=1  Side=Left
  connections:
  base_top_joint/RConn1 -- top_plate/LConn1
  Conn1/RConn1 -- base_top_joint/LConn1

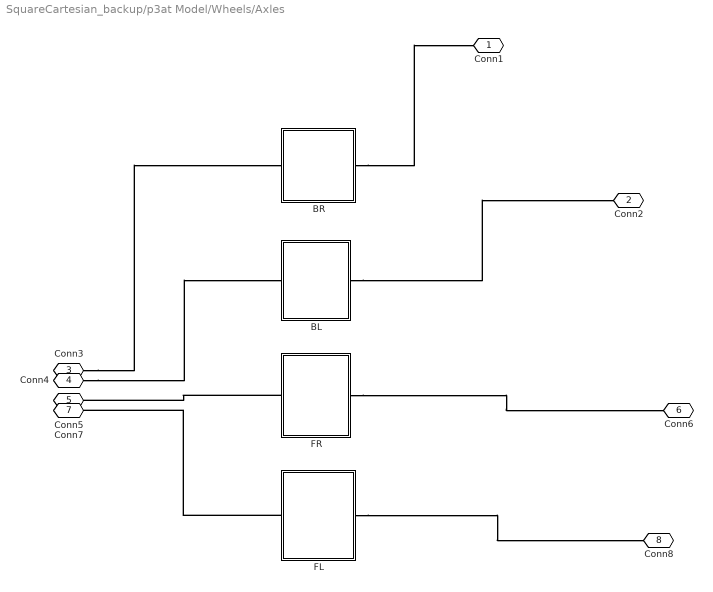
== system SquareCartesian_backup/p3at Model/Wheels/Axles ==
  BL : Subsystem
  BR : Subsystem
  FL : Subsystem
  FR : Subsystem
  Conn1 : PMIOPort  Port=1  Side=Right
  Conn2 : PMIOPort  Port=2  Side=Right
  Conn3 : PMIOPort  Port=3  Side=Left
  Conn4 : PMIOPort  Port=4  Side=Left
  Conn5 : PMIOPort  Port=5  Side=Left
  Conn6 : PMIOPort  Port=6  Side=Right
  Conn7 : PMIOPort  Port=7  Side=Left
  Conn8 : PMIOPort  Port=8  Side=Right
  connections:
  FR/RConn1 -- Conn6/RConn1
  FL/RConn1 -- Conn8/RConn1
  BR/RConn1 -- Conn1/RConn1
  BL/RConn1 -- Conn2/RConn1
  FL/LConn1 -- Conn7/RConn1
  Conn4/RConn1 -- BL/LConn1
  FR/LConn1 -- Conn5/RConn1
  Conn3/RConn1 -- BR/LConn1

== system SquareCartesian_backup/p3at Model/Wheels/Left Side ==
  In1 : Inport
  w_BL : Subsystem
  w_FL : Subsystem
  Conn1 : PMIOPort  Port=1  Side=Right
  Conn2 : PMIOPort  Port=2  Side=Right
  Conn3 : PMIOPort  Port=3  Side=Left
  Conn4 : PMIOPort  Port=4  Side=Left
  BL : Outport
  FL : Outport  Port=2
  wires:
  w_FL/1(w_FL_sensor) -> FL/1
  In1/1 -> w_BL/1(w_BL), w_FL/1(w_FL)
  w_BL/1(w_BL_sensor) -> BL/1
  connections:
  Conn4/RConn1 -- w_FL/LConn1
  w_FL/RConn1 -- Conn1/RConn1
  Conn2/RConn1 -- w_BL/RConn1
  Conn3/RConn1 -- w_BL/LConn1

== system SquareCartesian_backup/p3at Model/Wheels/Right Side ==
  In1 : Inport
  w_BR : Subsystem
  w_FR : Subsystem
  Conn1 : PMIOPort  Port=1  Side=Left
  Conn2 : PMIOPort  Port=2  Side=Right
  Conn3 : PMIOPort  Port=3  Side=Left
  Conn4 : PMIOPort  Port=4  Side=Right
  BR : Outport
  FR : Outport  Port=2
  wires:
  w_BR/1(w_BR_sensor) -> BR/1
  w_FR/1(w_FR_sensor) -> FR/1
  In1/1 -> w_FR/1(w_FR), w_BR/1(w_BR)
  connections:
  Conn3/RConn1 -- w_FR/LConn1
  Conn1/RConn1 -- w_BR/LConn1
  Conn4/RConn1 -- w_BR/RConn1
  Conn2/RConn1 -- w_FR/RConn1

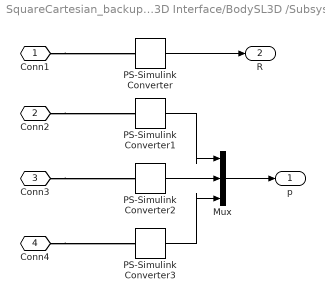
== system SquareCartesian_backup/Visual/SM-->SL3D Interface/BodySL3D /Subsystem ==
  Mux : Mux  Inputs=3
  PS-Simulink Converter{,1..3} (4 alike) : nesl_utility/PS-Simulink Converter  PhysicalDomain=network_engine_domain  SubClassName=ps_output  LeftPortType=input  RightPortType=output  PseudoPeriodic=off  Frequencies=[]  Unit=1  AffineConversion=off
  Conn1 : PMIOPort  Port=1  Side=Left
  Conn2 : PMIOPort  Port=2  Side=Left
  Conn3 : PMIOPort  Port=3  Side=Left
  Conn4 : PMIOPort  Port=4  Side=Left
  p : Outport
  R : Outport  Port=2
  wires:
  PS-Simulink Converter/1 -> R/1
  Mux/1 -> p/1
  PS-Simulink Converter1/1 -> Mux/1
  PS-Simulink Converter2/1 -> Mux/2
  PS-Simulink Converter3/1 -> Mux/3
  connections:
  Conn1/RConn1 -- PS-Simulink Converter/LConn1
  Conn3/RConn1 -- PS-Simulink Converter2/LConn1
  Conn4/RConn1 -- PS-Simulink Converter3/LConn1
  Conn2/RConn1 -- PS-Simulink Converter1/LConn1

== system SquareCartesian_backup/Visual/SM-->SL3D Interface/LWSL3D/Subsystem ==
  PS-Simulink Converter : nesl_utility/PS-Simulink Converter  PhysicalDomain=network_engine_domain  SubClassName=ps_output  LeftPortType=input  RightPortType=output  PseudoPeriodic=off  Frequencies=[]  Unit=1  AffineConversion=off
  Conn1 : PMIOPort  Port=1  Side=Left
  Omega_z : Outport
  wires:
  PS-Simulink Converter/1 -> Omega_z/1
  connections:
  Conn1/RConn1 -- PS-Simulink Converter/LConn1

== system SquareCartesian_backup/Visual/SM-->SL3D Interface/LWSL3D1/Subsystem ==
  PS-Simulink Converter : nesl_utility/PS-Simulink Converter  PhysicalDomain=network_engine_domain  SubClassName=ps_output  LeftPortType=input  RightPortType=output  PseudoPeriodic=off  Frequencies=[]  Unit=1  AffineConversion=off
  Conn1 : PMIOPort  Port=1  Side=Left
  Omega_z : Outport
  wires:
  PS-Simulink Converter/1 -> Omega_z/1
  connections:
  Conn1/RConn1 -- PS-Simulink Converter/LConn1

== system SquareCartesian_backup/Visual/SM-->SL3D Interface/RWSL3D/Subsystem ==
  PS-Simulink Converter : nesl_utility/PS-Simulink Converter  PhysicalDomain=network_engine_domain  SubClassName=ps_output  LeftPortType=input  RightPortType=output  PseudoPeriodic=off  Frequencies=[]  Unit=1  AffineConversion=off
  Conn1 : PMIOPort  Port=1  Side=Left
  Omega_z : Outport
  wires:
  PS-Simulink Converter/1 -> Omega_z/1
  connections:
  Conn1/RConn1 -- PS-Simulink Converter/LConn1

== system SquareCartesian_backup/Visual/SM-->SL3D Interface/RWSL3D1/Subsystem ==
  PS-Simulink Converter : nesl_utility/PS-Simulink Converter  PhysicalDomain=network_engine_domain  SubClassName=ps_output  LeftPortType=input  RightPortType=output  PseudoPeriodic=off  Frequencies=[]  Unit=1  AffineConversion=off
  Conn1 : PMIOPort  Port=1  Side=Left
  Omega_z : Outport
  wires:
  PS-Simulink Converter/1 -> Omega_z/1
  connections:
  Conn1/RConn1 -- PS-Simulink Converter/LConn1

== system SquareCartesian_backup/p3at Model/Fixed Bodies/Sonar Arrays/back_sonar ==
  Inertia : sm_lib/Body Elements/Solid  InertiaType=Custom  Mass=0.1  MassUnits=kg  CenterOfMass=[0, 0, 0]  CenterOfMassUnits=m  MomentsOfInertia=[1, 1, 1]  MomentsOfInertiaUnits=kg*m^2  ProductsOfInertia=[0, 0, 0]  ProductsOfInertiaUnits=kg*m^2  DensityBased=on  Density=1000  DensityUnits=kg/m^3  DoExposeReferenceFrame=on  SerializedFrames=<Frames/>  GraphicType=None  MarkerShape=Sphere  MarkerSize=10  GraphicVisPropType=SimpleVisualProperties  GraphicDiffuseColor=[0.5 0.5 0.5]  GraphicSpecularColor=[0.5 0.5 0.5 1.0]  GraphicAmbientColor=[0.15 0.15 0.15 1.0]  GraphicEmissiveColor=[0.0 0.0 0.0 1.0]  GraphicShininess=75  GraphicOpacity=1.0  GeometryShape=Sphere  RectangleSize=[1 1]  RectangleSizeUnits=m  BrickDimensions=[1 1 1]  BrickDimensionUnits=m  CylinderRadius=1  CylinderRadiusUnits=m  CylinderLength=1  CylinderLengthUnits=m  SphereRadius=1  SphereRadiusUnits=m  EllipsoidRadii=[1 1 1]  EllipsoidRadiiUnits=m  ExtrusionCrossSection=[1 1; -1 1; -1 -1; 1 -1]  ExtrusionCrossSectionUnits=m  ExtrusionLength=1  ExtrusionLengthUnits=m  PolygonNumSides=3  PolygonOuterRadius=1  PolygonOuterRadiusUnits=m  ExtGeomFileType=STEP  ExtGeomFileUnits=m  RevolutionCrossSection=[1 1; 1 -1; 2 -1; 2 1]  RevolutionCrossSectionUnits=m  RevolutionExtent=Full  RevolutionAngle=180  RevolutionAngleUnits=deg
  InertiaOriginTransform : sm_lib/Frames and Transforms/Rigid Transform  TranslationMethod=Cartesian  TranslationStandardOffset=0  TranslationLengthUnit=m  TranslationStandardAxis=+Z  TranslationCartesianOffset=[0, 0, 0]  TranslationROffset=0  TranslationROffsetUnits=m  TranslationZOffset=0  TranslationZOffsetUnits=m  TranslationThetaOffset=0  TranslationThetaOffsetUnits=deg  RotationMethod=RotationSequence  RotationAngleUnits=deg  RotationStandardAxis=+Z  RotationAngle=0.0  RotationArbitraryAxis=[0 0 1]  FollAlignAxisA=+X  BaseAlignAxisA=+Y  FollAlignAxisB=+Y  BaseAlignAxisB=+Z  RotationSequenceAxes=BaseAxes  RotationSequence=XYZ  RotationSequenceAngles=[0, 0, 0]  RotationSequenceAnglesUnits=rad  RotationMatrix=[1 0 0; 0 1 0; 0 0 1]
  ReferenceFrame : sm_lib/Frames and Transforms/Reference Frame
  Visual : sm_lib/Body Elements/Solid  InertiaType=Custom  Mass=0  MassUnits=kg  CenterOfMass=[0, 0, 0]  CenterOfMassUnits=m  MomentsOfInertia=[0, 0, 0]  MomentsOfInertiaUnits=kg*m^2  ProductsOfInertia=[0, 0, 0]  ProductsOfInertiaUnits=kg*m^2  DensityBased=on  Density=1000  DensityUnits=kg/m^3  DoExposeReferenceFrame=on  SerializedFrames=<Frames/>  GraphicType=FromGeometry  MarkerShape=Sphere  MarkerSize=10  GraphicVisPropType=SimpleVisualProperties  GraphicDiffuseColor=[0.715, 0.583, 0.21]  GraphicSpecularColor=[0.5 0.5 0.5 1.0]  GraphicAmbientColor=[0.15 0.15 0.15 1.0]  GraphicEmissiveColor=[0.0 0.0 0.0 1.0]  GraphicShininess=75  GraphicOpacity=1  GeometryShape=FromFile  RectangleSize=[1 1]  RectangleSizeUnits=m  BrickDimensions=[1 1 1]  BrickDimensionUnits=m  CylinderRadius=1  CylinderRadiusUnits=m  CylinderLength=1  CylinderLengthUnits=m  SphereRadius=1  SphereRadiusUnits=m  EllipsoidRadii=[1 1 1]  EllipsoidRadiiUnits=m  ExtrusionCrossSection=[1 1; -1 1; -1 -1; 1 -1]  ExtrusionCrossSectionUnits=m  ExtrusionLength=1  ExtrusionLengthUnits=m  PolygonNumSides=3  PolygonOuterRadius=1  PolygonOuterRadiusUnits=m  ExtGeomFileType=STL  ExtGeomFileName=/home/ty/catkin_ws/src/amr-ros-config/description/meshes/p3at_meshes/back_sonar.stl  ExtGeomFileUnits=m  RevolutionCrossSection=[1 1; 1 -1; 2 -1; 2 1]  RevolutionCrossSectionUnits=m  RevolutionExtent=Full  RevolutionAngle=180  RevolutionAngleUnits=deg
  VisualOriginTransform : sm_lib/Frames and Transforms/Rigid Transform  TranslationMethod=Cartesian  TranslationStandardOffset=0  TranslationLengthUnit=m  TranslationStandardAxis=+Z  TranslationCartesianOffset=[0, 0, 0]  TranslationROffset=0  TranslationROffsetUnits=m  TranslationZOffset=0  TranslationZOffsetUnits=m  TranslationThetaOffset=0  TranslationThetaOffsetUnits=deg  RotationMethod=RotationSequence  RotationAngleUnits=deg  RotationStandardAxis=+Z  RotationAngle=0.0  RotationArbitraryAxis=[0 0 1]  FollAlignAxisA=+X  BaseAlignAxisA=+Y  FollAlignAxisB=+Y  BaseAlignAxisB=+Z  RotationSequenceAxes=BaseAxes  RotationSequence=XYZ  RotationSequenceAngles=[0, 0, 0]  RotationSequenceAnglesUnits=rad  RotationMatrix=[1 0 0; 0 1 0; 0 0 1]
  F : PMIOPort  Port=1  Side=Left
  connections:
  Inertia/RConn1 -- InertiaOriginTransform/RConn1
  ReferenceFrame/RConn1 -- InertiaOriginTransform/LConn1 -- VisualOriginTransform/LConn1 -- F/RConn1
  Visual/RConn1 -- VisualOriginTransform/RConn1
